simulink model "FA_18_With_Controller"  (R2018a)
settings: Solver=ode45  StartTime=0.0  StopTime=200  RelTol=1e-3
PreLoadFcn:
  | F18_Linear
values from neighbouring files (symbols this model uses):
  C1 = [0 -1 0 1]    [F18_Linear.m]
  d2r = pi/180    (= 0.0174532925199)    [F18_Linear.m]    (also in FA_18_Trim.m; FA_18_sfun.m; Sim.m)
  F1 = [-67.81 11973 -133.3 -11801]    [F18_Linear.m]
  F2 = 1414.2    [F18_Linear.m]
  Trimx_N = [365.74;15*d2r;0;15*d2r]    [F18_Linear.m]
undefined symbols (not defined in the file or in its folder): Earth, WGS84
libraries: aerolibfltsims x1, aerolibtransform2 x1, aerolibconvert2 x1
settings Model: Creator=User  LastModifiedBy=User

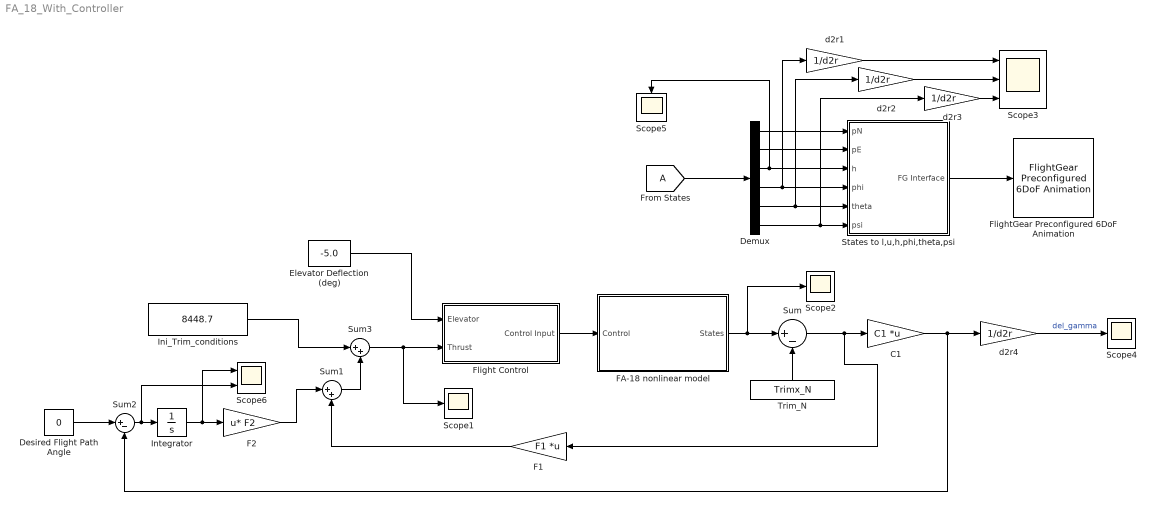
== system FA_18_With_Controller ==
  C1 : Gain  Gain=C1  Multiplication=Matrix(K*u)
  Demux : Demux  Outputs=6
  Desired Flight Path Angle : Constant  Value=0
  Elevator Deflection (deg) : Constant  Value=-5.0
  F1 : Gain  Gain=F1  Multiplication=Matrix(K*u)
  F2 : Gain  Gain=F2  Multiplication=Matrix(u*K)
  FA-18 nonlinear model : Subsystem
  Flight Control : Subsystem
  FlightGear Preconfigured 6DoF Animation : aerolibfltsims/FlightGear Preconfigured 6DoF Animation  xFlightGearVersion=v2017.3  DestinationIpAddress=127.0.0.1  DestinationPort=5502  SampleTime=1/30
      settings: SourceProductName=Aerospace Blockset
  Ini_Trim_conditions : Constant  Value=8448.7
  Integrator : Integrator
  Scope{1..2,4..5} (4 alike) : Scope
  Scope3 : Scope  NumInputPorts=3
  Scope6 : Scope  NumInputPorts=2
  States to l,u,h,phi,theta,psi : Subsystem
  Sum : Sum  Inputs=|+-
  Sum1 : Sum  Inputs=|++
  Sum2 : Sum  Inputs=|+-
  Sum3 : Sum  Inputs=|++
  Trim_N : Constant  Value=Trimx_N
  d2r{1..4} (4 alike) : Gain  Gain=1/d2r
  wires:
  Flight Control/1(Control Input) -> FA-18 nonlinear model/1(Control)
  Elevator Deflection (deg)/1 -> Flight Control/1(Elevator)
  FA-18 nonlinear model/1(States) -> Scope2/1, Sum/1
  Trim_N/1 -> Sum/2
  d2r4/1 -> Scope4/1  "del_gamma"
  Sum2/1 -> Scope6/2, Integrator/1
  Integrator/1 -> Scope6/1, F2/1
  Desired Flight Path Angle/1 -> Sum2/1
  C1/1 -> d2r4/1, Sum2/2
  F2/1 -> Sum1/1
  Sum1/1 -> Sum3/2
  F1/1 -> Sum1/2
  Sum3/1 -> Scope1/1, Flight Control/2(Thrust)
  Ini_Trim_conditions/1 -> Sum3/1
  Sum/1 -> F1/1, C1/1
  States to l,u,h,phi,theta,psi/1(FG Interface) -> FlightGear Preconfigured 6DoF Animation/1
  [A] -> Demux/1
  Demux/1 -> States to l,u,h,phi,theta,psi/1(pN)
  Demux/2 -> States to l,u,h,phi,theta,psi/2(pE)
  Demux/5 -> States to l,u,h,phi,theta,psi/5(theta), d2r2/1
  Demux/6 -> d2r3/1, States to l,u,h,phi,theta,psi/6(psi)
  Demux/4 -> d2r1/1, States to l,u,h,phi,theta,psi/4(phi)
  d2r1/1 -> Scope3/1
  d2r2/1 -> Scope3/2
  d2r3/1 -> Scope3/3
  Demux/3 -> Scope5/1, States to l,u,h,phi,theta,psi/3(h)

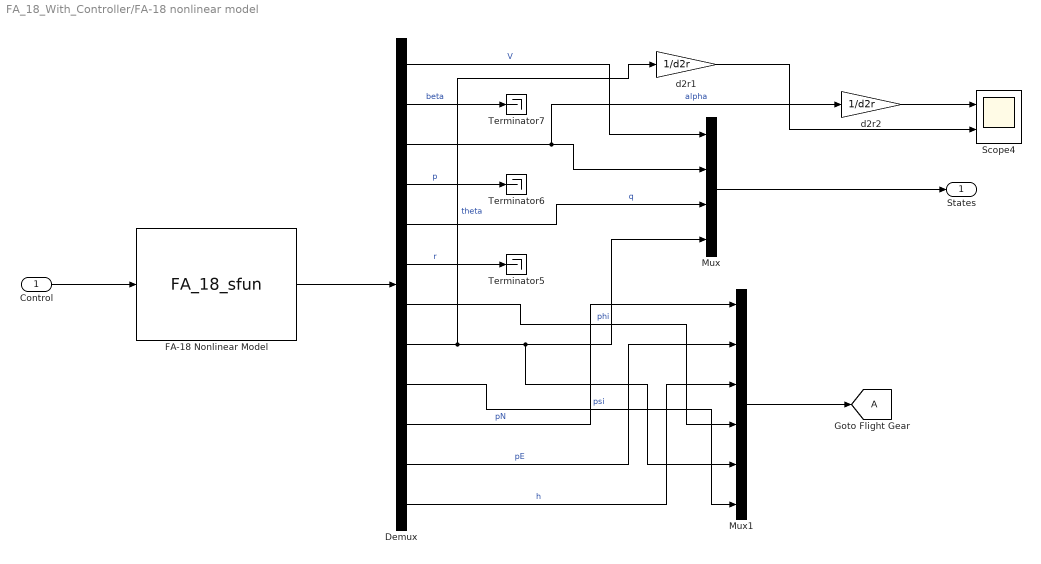
== system FA_18_With_Controller/FA-18 nonlinear model ==
  Control : Inport
  Demux : Demux  Outputs=12
  FA-18 Nonlinear Model : S-Function  FunctionName=FA_18_sfun  SFunctionDeploymentMode=off  EnableBusSupport=off
  Mux : Mux
  Mux1 : Mux  Inputs=6
  Scope4 : Scope  NumInputPorts=2
  Terminator5 : Terminator
  Terminator6 : Terminator
  Terminator7 : Terminator
  d2r1 : Gain  Gain=1/d2r
  d2r2 : Gain  Gain=1/d2r
  States : Outport
  tag scope: A=global
  wires:
  Control/1 -> FA-18 Nonlinear Model/1
  Demux/1 -> Mux/1  "V"
  FA-18 Nonlinear Model/1 -> Demux/1
  Demux/3 -> d2r2/1, Mux/2  "alpha"
  Demux/8 -> Mux1/5, Mux/4, d2r1/1  "theta"
  Demux/12 -> Mux1/3  "h"
  Demux/9 -> Mux1/6  "psi"
  Demux/11 -> Mux1/2  "pE"
  Demux/2 -> Terminator7/1  "beta"
  Demux/10 -> Mux1/1  "pN"
  Demux/6 -> Terminator5/1  "r"
  Demux/5 -> Mux/3  "q"
  Mux/1 -> States/1
  Demux/4 -> Terminator6/1  "p"
  Mux1/1 -> [A]
  Demux/7 -> Mux1/4  "phi"
  d2r1/1 -> Scope4/2
  d2r2/1 -> Scope4/1

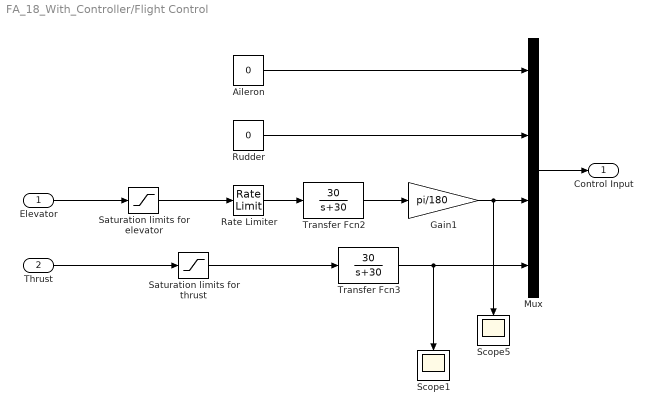
== system FA_18_With_Controller/Flight Control ==
  Elevator : Inport
  Thrust : Inport  Port=2
  Aileron : Constant  Value=0
  Gain1 : Gain  Gain=pi/180
  Mux : Mux
  Rate Limiter : RateLimiter  RisingSlewLimit=40  FallingSlewLimit=-40  SampleTimeMode=inherited
  Rudder : Constant  Value=0
  Saturation limits for elevator : Saturate  UpperLimit=10.5  LowerLimit=-24
  Saturation limits for thrust : Saturate  UpperLimit=20000  LowerLimit=0
  Scope1 : Scope
  Scope5 : Scope
  Transfer Fcn2 : TransferFcn  Numerator=[30]  Denominator=[1 30]
  Transfer Fcn3 : TransferFcn  Numerator=[30]  Denominator=[1 30]
  Control Input : Outport
  wires:
  Mux/1 -> Control Input/1
  Aileron/1 -> Mux/1
  Thrust/1 -> Saturation limits for thrust/1
  Transfer Fcn3/1 -> Scope1/1, Mux/4
  Rudder/1 -> Mux/2
  Saturation limits for thrust/1 -> Transfer Fcn3/1
  Saturation limits for elevator/1 -> Rate Limiter/1
  Rate Limiter/1 -> Transfer Fcn2/1
  Elevator/1 -> Saturation limits for elevator/1
  Gain1/1 -> Mux/3, Scope5/1
  Transfer Fcn2/1 -> Gain1/1

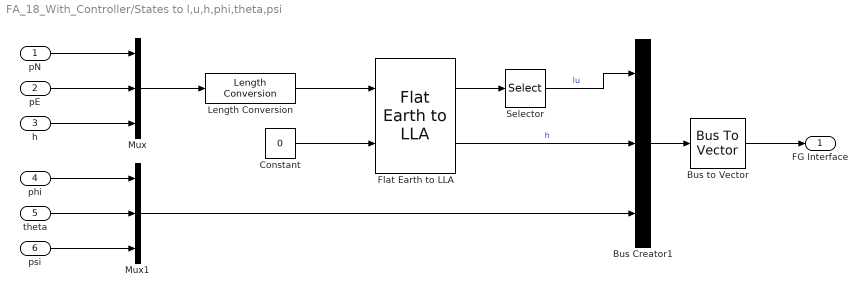
== system FA_18_With_Controller/States to l,u,h,phi,theta,psi ==
  pN : Inport
  pE : Inport  Port=2
  h : Inport  Port=3
  phi : Inport  Port=4
  theta : Inport  Port=5
  psi : Inport  Port=6
  Bus Creator1 : BusCreator  Inputs=3
  Bus to Vector : BusToVector
  Constant : Constant  Value=0
  Flat Earth to LLA : aerolibtransform2/Flat Earth to LLA  units=Metric (MKS)  ptype=Earth (WGS84)  F=1/298.257223563  R=6378137  LL0=[50.1018 14.2632]  psi=0
  Length Conversion : aerolibconvert2/Length Conversion  IU=ft  OU=m
  Mux : Mux  Inputs=3
  Mux1 : Mux  Inputs=3
  Selector : Selector  IndexMode=Zero-based  InputPortWidth=2  IndexOptions=Index vector (dialog)  Indices=[1 0]  OutputSizes=1
  FG Interface : Outport
  wires:
  Constant/1 -> Flat Earth to LLA/2
  Length Conversion/1 -> Flat Earth to LLA/1
  Bus to Vector/1 -> FG Interface/1
  Bus Creator1/1 -> Bus to Vector/1
  Flat Earth to LLA/1 -> Selector/1
  Selector/1 -> Bus Creator1/1  "lu"
  Flat Earth to LLA/2 -> Bus Creator1/2  "h"
  pN/1 -> Mux/1
  pE/1 -> Mux/2
  h/1 -> Mux/3
  Mux/1 -> Length Conversion/1
  theta/1 -> Mux1/2
  phi/1 -> Mux1/1
  psi/1 -> Mux1/3
  Mux1/1 -> Bus Creator1/3
